simulink model "dq0_modelling"  (R2025a)
settings: Solver=VariableStepAuto  StartTime=0.0  StopTime=0.1  MaxStep=1e-6  RelTol=1e-3
libraries: mcbeeMathTransformLib x2, spspowerguiLib x1
settings Model: Creator=prajw  LastModifiedBy=prajw

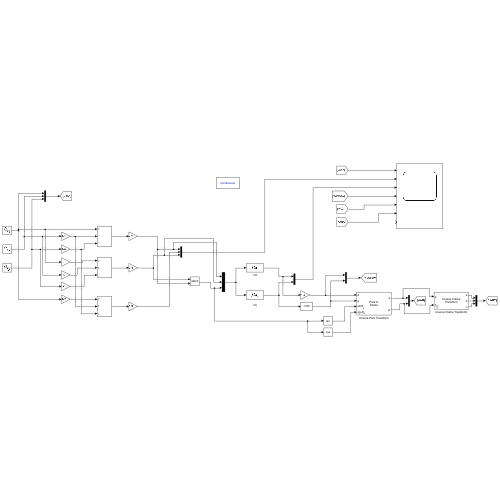
[thumbnail: Simulink's stored preview of the top-level diagram]
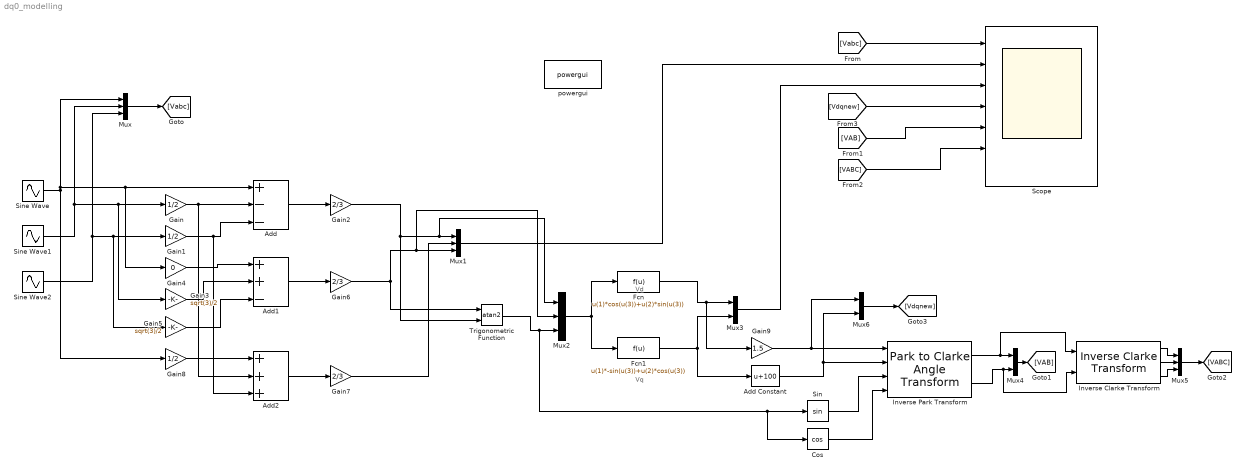
== system dq0_modelling ==
  note: Vq
  note: Vd
  Add : Sum  Inputs=+--
  Add Constant : Bias  Bias=100  SaturateOnIntegerOverflow=off
  Add1 : Sum  Inputs=++-
  Add2 : Sum  Inputs=+++
  Cos : Trigonometry  Operator=cos
  Fcn : Fcn  Expr=u(1)*cos(u(3))+u(2)*sin(u(3))
  Fcn1 : Fcn  Expr=u(1)*-sin(u(3))+u(2)*cos(u(3))
  Gain : Gain  Gain=1/2
  Gain1 : Gain  Gain=1/2
  Gain2 : Gain  Gain=2/3
  Gain3 : Gain  Gain=sqrt(3)/2
  Gain4 : Gain  Gain=0
  Gain5 : Gain  Gain=sqrt(3)/2
  Gain6 : Gain  Gain=2/3
  Gain7 : Gain  Gain=2/3
  Gain8 : Gain  Gain=1/2
  Gain9 : Gain  Gain=1.5
  Inverse Clarke Transform : mcbeeMathTransformLib/Inverse Clarke Transform  PowerInvariant=off  UseWithEmbedded=on  PhaseInput=Two inputs
      settings: LibrarySourceBlock=mcbhdllib/Controls/Math Transforms/Inverse Clarke Transform
  Inverse Park Transform : mcbeeMathTransformLib/Park to Clarke Angle Transform  AxisAlignment=D-axis  UseWithEmbedded=on  PhaseInput=Two inputs  ThetaInput=Sine and Cosine electrical position  AngleInput=Per-unit  N_points=1024
      settings: LibrarySourceBlock=mcbhdllib/Controls/Math Transforms/Inverse Park Transform
  Mux{,1..2,5} (4 alike) : Mux  Inputs=3
  Mux3 : Mux  Inputs=2
  Mux4 : Mux  Inputs=2
  Mux6 : Mux  Inputs=2
  Scope : Scope  NumInputPorts=7
      settings: ActiveDisplayString=6  ActiveDisplayYMinimum=-609.87959877339767  ActiveDisplayYMaximum=609.87959877339767  YLabel=Va'b'c'
  Sin : Trigonometry
  Sine Wave : Sin  Amplitude=230*sqrt(2)  Frequency=2*pi*50  SampleTime=0
  Sine Wave1 : Sin  Amplitude=230*sqrt(2)  Frequency=2*pi*50  Phase=2*pi/3  SampleTime=0
  Sine Wave2 : Sin  Amplitude=230*sqrt(2)  Frequency=2*pi*50  Phase=-2*pi/3  SampleTime=0
  Trigonometric Function : Trigonometry  Operator=atan2
  powergui : spspowerguiLib/powergui  Priority=1  SimulationMode=Continuous  SampleTime=50e-6  frequency=60  Iterations=50  frequencyindice=60  Pbase=100e6  ErrMax=1e-4  UnitsV=kV  UnitsW=MW  buscounter=0  FunctionMessages=off  echomessages=off  EnableUseOfTLC=off  CurrentSourceSwitches=off  DisableSnubberDevices=off  DisableRonSwitches=off  DisableVfSwitches=off  DisplayEquations=off  AutomaticDiscreteSolvers=off  SolverType=Tustin/Backward Euler (TBE)  Interpol=off  ExternalGateDelay=off  methode=off  Ts=100  x0status=blocks  SPID=on  SwTol=0  HookPort=off  NonlinearTolerance=1e-4  nMaxIteration=100  ContinueOnMaxIteration=off  RestoreLinks=warning  ResistiveCurrentMeasurement=off  Frange=[0:2:500]  Ylog=off  Xlog=on  ShowGrid=off  save=off  variable=ZData  structure=0  ZoomFFT=off  StartTime=0.0  cycles=1  DisplayStyle=1  fundamental=60  FreqAxis=off  MaxFrequency=1000  frequencyindicesteady=1  RmsSteady=1  display=off
  wires:
  Sine Wave/1 -> Gain4/1, Add/1, Mux/1, Gain8/1
  Sine Wave1/1 -> Gain3/1, Gain/1, Mux/2
  Sine Wave2/1 -> Gain5/1, Gain1/1, Mux/3
  Mux/1 -> [Vabc]
  [Vabc] -> Scope/1
  Gain/1 -> Add2/2, Add/2
  Gain1/1 -> Add2/3, Add/3
  Add/1 -> Gain2/1
  Gain2/1 -> Trigonometric Function/2, Mux2/1, Mux1/1
  Gain4/1 -> Add1/1
  Gain5/1 -> Add1/3
  Gain3/1 -> Add1/2
  Add1/1 -> Gain6/1
  Gain6/1 -> Trigonometric Function/1, Mux2/2, Mux1/3
  Mux1/1 -> Scope/2
  Add2/1 -> Gain7/1
  Gain7/1 -> Mux1/2
  Gain8/1 -> Add2/1
  Trigonometric Function/1 -> Cos/1, Sin/1, Mux2/3
  Mux2/1 -> Fcn1/1, Fcn/1
  Fcn1/1 -> Add Constant/1, Mux3/2
  Fcn/1 -> Mux3/1, Gain9/1
  Mux3/1 -> Scope/3
  Add Constant/1 -> Mux6/2, Inverse Park Transform/2
  Gain9/1 -> Mux6/1, Inverse Park Transform/1
  Sin/1 -> Inverse Park Transform/3
  Cos/1 -> Inverse Park Transform/4
  Inverse Park Transform/1 -> Inverse Clarke Transform/1, Mux4/1
  Inverse Park Transform/2 -> Inverse Clarke Transform/2, Mux4/2
  Mux4/1 -> [VAB]
  [VAB] -> Scope/5
  Inverse Clarke Transform/1 -> Mux5/1
  Inverse Clarke Transform/2 -> Mux5/2
  Inverse Clarke Transform/3 -> Mux5/3
  Mux5/1 -> [VABC]
  [VABC] -> Scope/6
  Mux6/1 -> [Vdqnew]
  [Vdqnew] -> Scope/4
